simulink model "sensor_model"  (R2025b)
settings: Solver=FixedStepDiscrete  StartTime=0.0  StopTime=10.0  FixedStep=0.001  RelTol=1e-3
settings Model: DataDictionary=SensorDict.sldd  Creator=89447  LastModifiedBy=89447

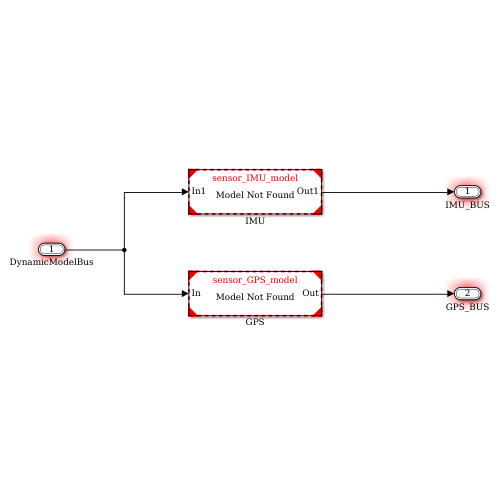
[thumbnail: Simulink's stored preview of the top-level diagram]
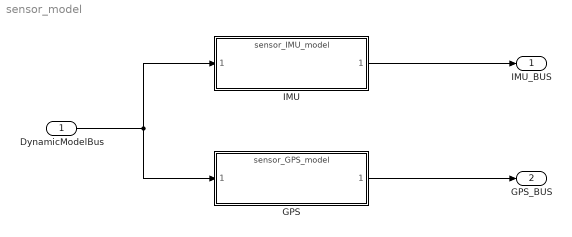
== system sensor_model ==
  DynamicModelBus : Inport  OutDataTypeStr=Bus: DynamicModelBus
  GPS : ModelReference  ModelNameDialog=sensor_GPS_model.slx  SimulationMode=Normal  ModelReferenceVersion=4.4
  IMU : ModelReference  ModelNameDialog=sensor_IMU_model.slx  SimulationMode=Normal  ModelReferenceVersion=4.7
  IMU_BUS : Outport  OutDataTypeStr=Bus: IMU_BUS
  GPS_BUS : Outport  Port=2  OutDataTypeStr=Bus: GPS_BUS
  wires:
  DynamicModelBus/1 -> GPS/1, IMU/1
  IMU/1 -> IMU_BUS/1
  GPS/1 -> GPS_BUS/1
